simulink model "sim_battery_system"  (R2018b)
settings: Solver=FixedStepDiscrete  StartTime=0.0  StopTime=SimPara.t_sim  FixedStep=SimPara.t_step  RelTol=1e-3
undefined symbols (not defined in the file or in its folder): A, BatPara, i, LSAPara, p, SimPara, SysPara, x2_cal, x3_cal, x_cal
libraries: simulink x14, dspstat3 x4, dspindex x1
(part 1 of 4)
Description:
  | A simulation framework for lithium-ion battery systems.
  | Refer to https://github.com/TUMFTM/sim_battery_system for futher information.
  | 
  | Authors:
  | 
  | Christoph Reiter (christoph.reiter@tum.de)
  | Johannes Dirnecker
  | Leo Wildfeuer
  | André Thomaser
  | Thilo Krahl
  | Sebastian Huber
  | Thilo Wurster
  | 
  | Created at:
  | 
  | Institute of Automotive Technology
  | Department of Mechanical Engineering
  | Technical University of Munich
settings Model: SimulationMode=accelerator  NumberOfSteps=300  Creator=Christoph Reiter  LastModifiedBy=gu74niw
settings SolverCC: AutoInsertRateTranBlk=on  InsertRTBMode=Always
settings DataIOCC: LimitDataPoints=on  MaxDataPoints=1  SaveFormat=Structure  SaveOutput=off  SignalLogging=off  DSMLogging=off  SaveTime=off
settings OptimizationCC: DefaultParameterBehavior=Inlined  UseFloatMulNetSlope=on  InlineInvariantSignals=on  EfficientFloat2IntCast=on  LifeSpan=inf
settings DebuggingCC: ReadBeforeWriteMsg=DisableAll  WriteAfterWriteMsg=DisableAll  WriteAfterReadMsg=DisableAll  AlgebraicLoopMsg=error  SaveWithParameterizedLinksMsg=none  UnderspecifiedInitializationDetection=Classic  MultiTaskDSMMsg=none  MultiTaskCondExecSysMsg=warning  MultiTaskRateTransMsg=warning  SingleTaskRateTransMsg=warning  UniqueDataStoreMsg=error  AllowSymbolicDim=off  StrictBusMsg=ErrorOnBusTreatedAsVector  SFUnexpectedBacktrackingDiag=warning  SFNoUnconditionalDefaultTransitionDiag=warning  SFExecutionAtInitializationDiag=none
settings HardwareCC: ProdBitPerPointer=32  ProdBitPerSizeT=32  ProdBitPerPtrDiffT=32  ProdLargestAtomicFloat=None  ProdIntDivRoundTo=Undefined  ProdEndianess=Unspecified  ProdWordSize=32  ProdHWDeviceType=32-bit Generic  TargetBitPerPointer=64  TargetBitPerSizeT=64  TargetBitPerPtrDiffT=64  TargetLongLongMode=on  TargetIntDivRoundTo=Zero  TargetEndianess=LittleEndian  TargetWordSize=64  TargetHWDeviceType=MATLAB Host
settings ModelReferenceCC: UpdateModelReferenceTargets=IfOutOfDate  EnableParallelModelReferenceBuilds=on  ParallelModelReferenceMATLABWorkerInit=Load Top Model  PropagateSignalLabelsOutOfModel=off
settings SFSimCC: SFSimEcho=off  SimUseLocalCustomCode=off
settings RTWCC: RTWUseLocalCustomCode=off  Toolchain=Microsoft Visual C++ 2015 v14.0 | nmake (64-bit Windows)  BuildConfiguration=Faster Runs
settings CodeAppCC: ForceParamTrailComments=on  StateflowObjectComments=on  MATLABSourceComments=on
settings GRTTargetCC: GeneratePreprocessorConditionals=Disable all  MatFileLogging=off  SupportNonFinite=off
settings ConfigComp: CovMetricSettings=dw  CovHtmlReporting=on  CovSaveCumulativeToWorkspaceVar=on  CovSaveSingleToWorkspaceVar=on  CovExternalEMLEnable=off  CovSFcnEnable=off

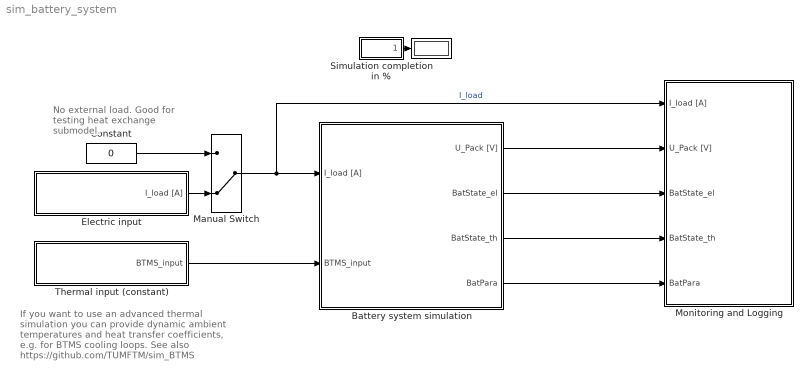
== system sim_battery_system ==
  note: No external load. Good for
      | testing heat exchange submodel.
  note: If you want to use an advanced thermal simulation
      | you can provide dynamic ambient temperatures
      | and heat transfer coefficients, e.g. for BTMS cooling
      | loops.
      | See also https://github.com/TUMFTM/sim_BTMS
  "\t\t      Simulation completion in %\t" : Subsystem
  " " : Display
      settings: Format=bank
  Battery system simulation : Subsystem  TreatAsAtomicUnit=on
  Constant : Constant  Value=0
  Electric input : Subsystem
  Manual Switch : ManualSwitch  CurrentSetting=0
  Monitoring and Logging : Subsystem
  Thermal input (constant) : Subsystem
  wires:
  "\t\t      Simulation completion in %\t"/1(" ") -> " "/1
  Manual Switch/1 -> Monitoring and Logging/1(I_load [A]), Battery system simulation/1(I_load [A])  "I_load"
  Thermal input (constant)/1(BTMS_input) -> Battery system simulation/2(BTMS_input)
  Battery system simulation/1(U_Pack [V]) -> Monitoring and Logging/2(U_Pack [V])
  Battery system simulation/2(BatState_el) -> Monitoring and Logging/3(BatState_el)
  Battery system simulation/3(BatState_th) -> Monitoring and Logging/4(BatState_th)
  Battery system simulation/4(BatPara) -> Monitoring and Logging/5(BatPara)
  Electric input/1(I_load [A]) -> Manual Switch/2
  Constant/1 -> Manual Switch/1

== system sim_battery_system/		      Simulation completion in %	 ==
  note: Determine simulation completion
  Clock : Clock
  Divide : Product  Inputs=*/
  max. Simulaton Time : Constant  Value=SimPara.t_sim
  to % : Gain  Gain=100
  " " : Outport
  wires:
  max. Simulaton Time/1 -> Divide/2
  Clock/1 -> Divide/1
  Divide/1 -> to %/1
  to %/1 -> " "/1

== system sim_battery_system/Battery system simulation ==
  I_load [A] : Inport
  BTMS_input : Inport  Port=2
  Electrical Submodel : Subsystem
  Save BatState_el of last time-step : Subsystem
  Save BatState_th of last time-step : Subsystem
  Static and dynamic LIB parameters : Subsystem
  Thermal Submodel : Subsystem
  U_Pack [V] : Outport
  BatState_el : Outport  Port=2
  BatState_th : Outport  Port=3
  BatPara : Outport  Port=4
  wires:
  Static and dynamic LIB parameters/1(BatPara) -> Electrical Submodel/2(BatPara), Thermal Submodel/4(BatPara), BatPara/1
  Electrical Submodel/1(BatState_el) -> BatState_el/1, Save BatState_el of last time-step/1(BatState_el), Thermal Submodel/3(BatState_el)
  I_load [A]/1 -> Electrical Submodel/1(I_Pack [A])
  Electrical Submodel/2(U_Pack [V]) -> U_Pack [V]/1
  Save BatState_el of last time-step/1(BatState_el_in) -> Static and dynamic LIB parameters/2(BatState_el_in), Electrical Submodel/3(BatState_in)
  Thermal Submodel/1(BatState_th) -> BatState_th/1, Save BatState_th of last time-step/1(BatState_th)
  Save BatState_th of last time-step/1(Bat_State_th_in) -> Thermal Submodel/1(BatState_th_in), Static and dynamic LIB parameters/1(BatState_th_in)
  BTMS_input/1 -> Thermal Submodel/2(BTMS_input)

== system sim_battery_system/Electric input ==
  note: Dummy load cycle. Scaled from cell measurement, so U_terminal
      | has nothing to do with the battery system you may specify.
  Demux : Demux  Outputs=2
  From Workspace : FromWorkspace  VariableName=load_cycle  SampleTime=0  OutputAfterFinalValue=Setting to zero
  Terminator : Terminator
  I_load [A] : Outport  Unit=A
  wires:
  From Workspace/1 -> Demux/1
  Demux/1 -> Terminator/1  "U_terminal"
  Demux/2 -> I_load [A]/1  "I_load"

== system sim_battery_system/Monitoring and Logging ==
  I_load [A] : Inport
  U_Pack [V] : Inport  Port=2
  BatState_el : Inport  Port=3
  BatState_th : Inport  Port=4
  BatPara : Inport  Port=5
  Constant : Constant  Value=SimPara.LoggingOutput
  Load Spectrum Analysis : Subsystem  Variant=on  VariantControl=Variant1
  Logging of Variables : Subsystem
  Temperature Sensor Simulation : Subsystem
  wires:
  I_load [A]/1 -> Logging of Variables/1(I_load [A])
  U_Pack [V]/1 -> Logging of Variables/2(U_Pack [A])
  BatState_el/1 -> Logging of Variables/3(BatState_el), Load Spectrum Analysis/1("BatState_el ")
  BatState_th/1 -> Temperature Sensor Simulation/1(bat_state_th_in)
  BatPara/1 -> Load Spectrum Analysis/3("BatPara ")
  Constant/1 -> Logging of Variables/Enable
  Temperature Sensor Simulation/1(bat_state_th_out) -> Load Spectrum Analysis/2("BatState_th ")

== system sim_battery_system/Thermal input (constant) ==
  Bus Creator : BusCreator  Inputs=2
  Constant : Constant  Value=SysPara.thermal.T_cell_ambient
  Constant1 : Constant  Value=SysPara.thermal.alpha_cell_ambient
  BTMS_input : Outport
  wires:
  Constant1/1 -> Bus Creator/2  "alpha_cell_ambient"
  Constant/1 -> Bus Creator/1  "T_cell_ambient"
  Bus Creator/1 -> BTMS_input/1  "BTMS_input"

== system sim_battery_system/Battery system simulation/Electrical Submodel ==
  note: Delay resulting balancing current for one step to avoid algebraic loop
  I_Pack [A] : Inport
  BatPara : Inport  Port=2
  BatState_in : Inport  Port=3
  Bus Creator1 : BusCreator  Inputs=8
  Cell Balancing : Subsystem
  Electric potential (single cell) : Subsystem
  Ohmic voltage drop and compensating currents in parallel connections : Subsystem
  Unit Delay4 : UnitDelay  InitialCondition=zeros(SysPara.p,SysPara.s)  SampleTime=-1
  Voltage of battery system : Subsystem
  dt : Subsystem
  BatState_el : Outport
  U_Pack [V] : Outport  Port=2
  wires:
  I_Pack [A]/1 -> Cell Balancing/1(I_Pack [A]), Ohmic voltage drop and compensating currents in parallel connections/2(I_Pack [A])
  Unit Delay4/1 -> Ohmic voltage drop and compensating currents in parallel connections/1(I_Balancing_in [A])  "I_Balancing_in [A]"
  Ohmic voltage drop and compensating currents in parallel connections/1(U_Cell [V]) -> Bus Creator1/1, Voltage of battery system/1(U_Cells [V]), Cell Balancing/2(U_Cell [V])
  Ohmic voltage drop and compensating currents in parallel connections/2(I_Cell [A]) -> Bus Creator1/2
  Ohmic voltage drop and compensating currents in parallel connections/3(U_R [V]) -> Bus Creator1/3
  Cell Balancing/1(I_Balancing [A]) -> Unit Delay4/1
  Voltage of battery system/1(U_Pack [V]) -> U_Pack [V]/1
  Bus Creator1/1 -> BatState_el/1  "BatState_el"
  BatPara/1 -> Ohmic voltage drop and compensating currents in parallel connections/3(BatPara), Electric potential (single cell)/1(BatPara)
  Electric potential (single cell)/1(U_Potential) -> Ohmic voltage drop and compensating currents in parallel connections/4(U_Potential [V]), Bus Creator1/4
  dt/1(dt [s]) -> Electric potential (single cell)/2(dt)
  BatState_in/1 -> Electric potential (single cell)/3(BatState_in)
  Electric potential (single cell)/2(SOC) -> Bus Creator1/5
  Electric potential (single cell)/3(U_OCV) -> Bus Creator1/6
  Electric potential (single cell)/4(U_Hysteresis) -> Bus Creator1/7
  Electric potential (single cell)/5(U_RC) -> Bus Creator1/8

== system sim_battery_system/Battery system simulation/Save BatState_el of last time-step ==
  note: Delay system state variables by one step to avoid algebraic loop.
      | We need these for the parameter lookup-tables
  BatState_el : Inport
  Bus Creator : BusCreator  Inputs=4
  Bus Creator2 : BusCreator  Inputs=4
  Bus Selector : BusSelector  OutputSignals=U_RC1 [V],U_RC2 [V],U_RC3 [V],U_RC4 [V]
  Bus Selector1 : BusSelector  OutputSignals=SOC,U_Hysteresis [V],I_cell [A],U_RC [V]
  Unit Delay : UnitDelay  InitialCondition=SysPara.BatStateInit.electrical.SOC  SampleTime=-1
  Unit Delay1 : UnitDelay  InitialCondition=SysPara.BatStateInit.electrical.U_hyst  SampleTime=-1
  Unit Delay2 : UnitDelay  InitialCondition=SysPara.BatStateInit.electrical.U_RC1  SampleTime=-1
  Unit Delay3 : UnitDelay  InitialCondition=SysPara.BatStateInit.electrical.U_RC2  SampleTime=-1
  Unit Delay4 : UnitDelay  InitialCondition=SysPara.BatStateInit.electrical.I_cell  SampleTime=-1
  Unit Delay5 : UnitDelay  InitialCondition=SysPara.BatStateInit.electrical.U_RC3  SampleTime=-1
  Unit Delay6 : UnitDelay  InitialCondition=SysPara.BatStateInit.electrical.U_RC4  SampleTime=-1
  BatState_el_in : Outport
  wires:
  Bus Selector1/2 -> Unit Delay1/1  "<U_Hysteresis [V]>"
  Unit Delay4/1 -> Bus Creator2/3  "I_cell [A]"
  Bus Selector1/3 -> Unit Delay4/1  "<I_cell [A]>"
  Unit Delay1/1 -> Bus Creator2/2  "U_Hysteresis [V]"
  Bus Selector1/1 -> Unit Delay/1  "<SOC>"
  Unit Delay/1 -> Bus Creator2/1  "SOC"
  Bus Creator2/1 -> BatState_el_in/1  "BatState_el_in"
  BatState_el/1 -> Bus Selector1/1
  Bus Selector1/4 -> Bus Selector/1  "<U_RC [V]>"
  Bus Selector/1 -> Unit Delay2/1  "<U_RC1 [V]>"
  Bus Selector/2 -> Unit Delay3/1  "<U_RC2 [V]>"
  Bus Selector/3 -> Unit Delay5/1  "<U_RC3 [V]>"
  Bus Selector/4 -> Unit Delay6/1  "<U_RC4 [V]>"
  Unit Delay6/1 -> Bus Creator/4  "U_RC4 [V]"
  Unit Delay5/1 -> Bus Creator/3  "U_RC3 [V]"
  Unit Delay3/1 -> Bus Creator/2  "U_RC2 [V]"
  Unit Delay2/1 -> Bus Creator/1  "U_RC1 [V]"
  Bus Creator/1 -> Bus Creator2/4  "U_RC"

== system sim_battery_system/Battery system simulation/Save BatState_th of last time-step ==
  note: Delay system state variables by one step to avoid algebraic loop.
      | We need these for the parameter lookup-tables
  BatState_th : Inport
  Bus Creator1 : BusCreator  Inputs=1
  Bus Selector : BusSelector  OutputSignals=T_cell [°C]
  Unit Delay1 : UnitDelay  InitialCondition=SysPara.BatStateInit.thermal.T_cell  SampleTime=-1
  Bat_State_th_in : Outport
  wires:
  Unit Delay1/1 -> Bus Creator1/1  "T_cell [°C]"
  Bus Selector/1 -> Unit Delay1/1  "<T_cell [°C]>"
  Bus Creator1/1 -> Bat_State_th_in/1  "Bat_State_th_in"
  BatState_th/1 -> Bus Selector/1

== system sim_battery_system/Battery system simulation/Static and dynamic LIB parameters ==
  BatState_th_in : Inport
  BatState_el_in : Inport  Port=2
  LIB Parameter Look-Ups : Subsystem
  Statistic Cell Deviations : Subsystem
  BatPara : Outport
  wires:
  LIB Parameter Look-Ups/1(BatPara_el_uniform) -> Statistic Cell Deviations/1("BatPara_el_uniform ")
  Statistic Cell Deviations/1(BatPara) -> BatPara/1  "BatPara"
  BatState_el_in/1 -> LIB Parameter Look-Ups/2(BatState_el_in)
  BatState_th_in/1 -> LIB Parameter Look-Ups/1(BatState_th_in)

== system sim_battery_system/Battery system simulation/Thermal Submodel ==
  note: Total cell heat generation:
      |
      | PQ_cell = PQ_cell,irr + PQ_cell,rev
  BatState_th_in : Inport
  BTMS_input : Inport  Port=2
  BatState_el : Inport  Port=3
  BatPara : Inport  Port=4
  Add : Sum
  Bus Creator : BusCreator  Inputs=6
  Bus Selector : BusSelector  OutputSignals=U_R [V],U_RC [V],I_cell [A]
  Bus Selector3 : BusSelector  OutputSignals=alpha_cell_ambient,T_cell_ambient
  Bus Selector4 : BusSelector  OutputSignals=T_cell [°C]
  Cell heat transport and heat dissipation : Subsystem
  Constant : Constant  Value=SimPara.thermal_sim_enable
  Irreversible heat generation : Subsystem
  Reversible heat generation : Subsystem
  BatState_th : Outport
  wires:
  Bus Selector3/2 -> Cell heat transport and heat dissipation/5(T_cell_ambient), Bus Creator/5  "<T_cell_ambient>"
  Add/1 -> Cell heat transport and heat dissipation/1(PQ_cell), Bus Creator/1  "PQ_cell [W]"
  Bus Creator/1 -> BatState_th/1  "BatState_th"
  Bus Selector3/1 -> Cell heat transport and heat dissipation/4(alpha_cell_ambient), Bus Creator/6  "<alpha_cell_ambient>"
  Irreversible heat generation/1(PQ_cell,irr [W]) -> Add/1
  Reversible heat generation/1(PQ_cell,rev [W]) -> Add/2
  BatPara/1 -> Cell heat transport and heat dissipation/2(BatPara), Reversible heat generation/3(BatPara)
  BatState_el/1 -> Bus Selector/1
  Bus Selector/2 -> Irreversible heat generation/2(U_RC)  "<U_RC [V]>"
  Bus Selector/3 -> Reversible heat generation/1(I_Cells [A]), Irreversible heat generation/3(I_Cells [A])  "<I_cell [A]>"
  Bus Selector/1 -> Irreversible heat generation/1(U_R [V])  "<U_R [V]>"
  BTMS_input/1 -> Bus Selector3/1
  BatState_th_in/1 -> Bus Selector4/1
  Bus Selector4/1 -> Reversible heat generation/2(T_Cells [°C]), Cell heat transport and heat dissipation/3(T_cell_in)  "<T_cell [°C]>"
  Cell heat transport and heat dissipation/1(T_cell [°C]) -> Bus Creator/2
  Constant/1 -> Cell heat transport and heat dissipation/Enable
  Cell heat transport and heat dissipation/3(PQ_transfer [W]) -> Bus Creator/4
  Cell heat transport and heat dissipation/2(PQ_ambient [W]) -> Bus Creator/3

== system sim_battery_system/Monitoring and Logging/Load Spectrum Analysis ==
  "BatState_el " : Inport
  "BatState_th " : Inport  Port=2
  "BatPara " : Inport  Port=3
  Load Spectrum Analysis OFF : Subsystem  VariantControl=SimPara.LoadSpectra_enable == 0
  Load Spectrum Analysis ON : Subsystem  VariantControl=SimPara.LoadSpectra_enable == 1

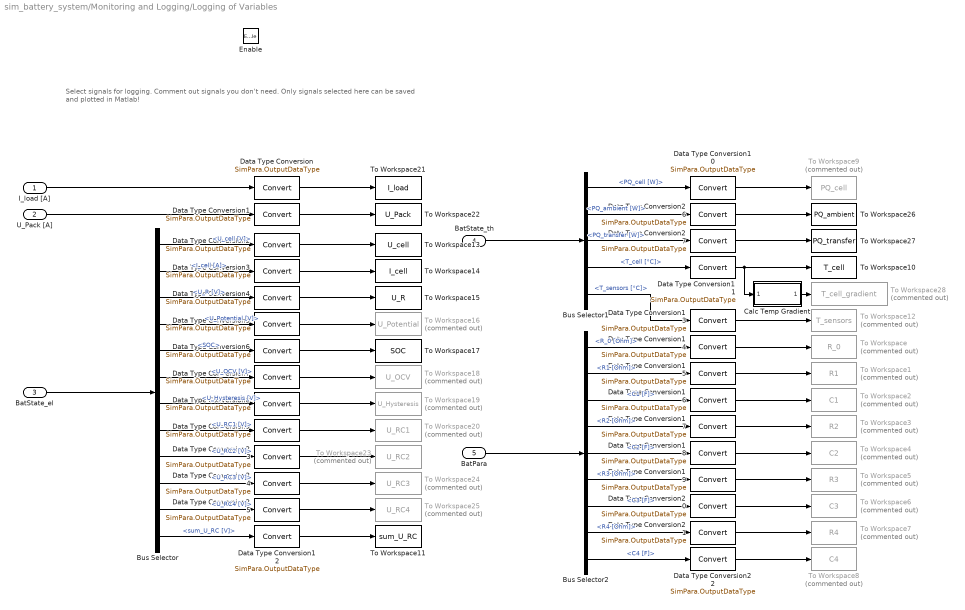
== system sim_battery_system/Monitoring and Logging/Logging of Variables ==
  note: Select signals for logging. Comment out signals you don't need.
      | Only signals selected here can be saved and plotted in Matlab!
  I_load [A] : Inport
  U_Pack [A] : Inport  Port=2
  BatState_el : Inport  Port=3
  BatState_th : Inport  Port=4
  BatPara : Inport  Port=5
  Enable : EnablePort
  Bus Selector : BusSelector  OutputSignals=U_cell [V],I_cell [A],U_R [V],U_Potential [V],SOC,U_OCV [V],U_Hysteresis [V],U_RC [V].U_RC1 [V],U_RC [V].U_RC2 [V],U_RC [V].U_RC3 [V],U_RC [V].U_RC4 [V],U_RC [V].sum_U_RC [V]
  Bus Selector1 : BusSelector  OutputSignals=PQ_cell [W],PQ_ambient [W],PQ_transfer [W],T_cell [°C],T_sensors [°C]
  Bus Selector2 : BusSelector  OutputSignals=electrical.R_0 [Ohm],electrical.R1 [Ohm],electrical.C1 [F],electrical.R2 [Ohm],electrical.C2 [F],electrical.R3 [Ohm],electrical.C3 [F],electrical.R4 [Ohm],electrical.C4 [F]
  Calc Temp Gradient : Subsystem
  Data Type Conversion{,1..27} (28 alike) : DataTypeConversion  OutDataTypeStr=SimPara.OutputDataType
  To Workspace : ToWorkspace  Commented=on  VariableName=R_0  SaveFormat=Timeseries  SampleTime=-1
      settings: Decimation=SimPara.OutputDecimation
  To Workspace1 : ToWorkspace  Commented=on  VariableName=R1  SaveFormat=Timeseries  SampleTime=-1
      settings: Decimation=SimPara.OutputDecimation
  To Workspace10 : ToWorkspace  VariableName=T_cell  SaveFormat=Timeseries  SampleTime=-1
      settings: Decimation=SimPara.OutputDecimation
  To Workspace11 : ToWorkspace  VariableName=sum_U_RC  SaveFormat=Timeseries  SampleTime=-1
      settings: Decimation=SimPara.OutputDecimation
  To Workspace12 : ToWorkspace  Commented=on  VariableName=T_sensors  SaveFormat=Timeseries  SampleTime=-1
      settings: Decimation=SimPara.OutputDecimation
  To Workspace13 : ToWorkspace  VariableName=U_cell  SaveFormat=Timeseries  SampleTime=-1
      settings: Decimation=SimPara.OutputDecimation
  To Workspace14 : ToWorkspace  VariableName=I_cell  SaveFormat=Timeseries  SampleTime=-1
      settings: Decimation=SimPara.OutputDecimation
  To Workspace15 : ToWorkspace  VariableName=U_R  SaveFormat=Timeseries  SampleTime=-1
      settings: Decimation=SimPara.OutputDecimation
  To Workspace16 : ToWorkspace  Commented=on  VariableName=U_Potential  SaveFormat=Timeseries  SampleTime=-1
      settings: Decimation=SimPara.OutputDecimation
  To Workspace17 : ToWorkspace  VariableName=SOC  SaveFormat=Timeseries  SampleTime=-1
      settings: Decimation=SimPara.OutputDecimation
  To Workspace18 : ToWorkspace  Commented=on  VariableName=U_OCV  SaveFormat=Timeseries  SampleTime=-1
      settings: Decimation=SimPara.OutputDecimation
  To Workspace19 : ToWorkspace  Commented=on  VariableName=U_Hysteresis  SaveFormat=Timeseries  SampleTime=-1
      settings: Decimation=SimPara.OutputDecimation
  To Workspace2 : ToWorkspace  Commented=on  VariableName=C1  SaveFormat=Timeseries  SampleTime=-1
      settings: Decimation=SimPara.OutputDecimation
  To Workspace20 : ToWorkspace  Commented=on  VariableName=U_RC1  SaveFormat=Timeseries  SampleTime=-1
      settings: Decimation=SimPara.OutputDecimation
  To Workspace21 : ToWorkspace  VariableName=I_load  SaveFormat=Timeseries  SampleTime=-1
      settings: Decimation=SimPara.OutputDecimation
  To Workspace22 : ToWorkspace  VariableName=U_Pack  SaveFormat=Timeseries  SampleTime=-1
      settings: Decimation=SimPara.OutputDecimation
  To Workspace23 : ToWorkspace  Commented=on  VariableName=U_RC2  SaveFormat=Timeseries  SampleTime=-1
      settings: Decimation=SimPara.OutputDecimation
  To Workspace24 : ToWorkspace  Commented=on  VariableName=U_RC3  SaveFormat=Timeseries  SampleTime=-1
      settings: Decimation=SimPara.OutputDecimation
  To Workspace25 : ToWorkspace  Commented=on  VariableName=U_RC4  SaveFormat=Timeseries  SampleTime=-1
      settings: Decimation=SimPara.OutputDecimation
  To Workspace26 : ToWorkspace  VariableName=PQ_ambient  SaveFormat=Timeseries  SampleTime=-1
      settings: Decimation=SimPara.OutputDecimation
  To Workspace27 : ToWorkspace  VariableName=PQ_transfer  SaveFormat=Timeseries  SampleTime=-1
      settings: Decimation=SimPara.OutputDecimation
  To Workspace28 : ToWorkspace  Commented=on  VariableName=T_cell_gradient  SaveFormat=Timeseries  SampleTime=-1
      settings: Decimation=SimPara.OutputDecimation
  To Workspace3 : ToWorkspace  Commented=on  VariableName=R2  SaveFormat=Timeseries  SampleTime=-1
      settings: Decimation=SimPara.OutputDecimation
  To Workspace4 : ToWorkspace  Commented=on  VariableName=C2  SaveFormat=Timeseries  SampleTime=-1
      settings: Decimation=SimPara.OutputDecimation
  To Workspace5 : ToWorkspace  Commented=on  VariableName=R3  SaveFormat=Timeseries  SampleTime=-1
      settings: Decimation=SimPara.OutputDecimation
  To Workspace6 : ToWorkspace  Commented=on  VariableName=C3  SaveFormat=Timeseries  SampleTime=-1
      settings: Decimation=SimPara.OutputDecimation
  To Workspace7 : ToWorkspace  Commented=on  VariableName=R4  SaveFormat=Timeseries  SampleTime=-1
      settings: Decimation=SimPara.OutputDecimation
  To Workspace8 : ToWorkspace  Commented=on  VariableName=C4  SaveFormat=Timeseries  SampleTime=-1
      settings: Decimation=SimPara.OutputDecimation
  To Workspace9 : ToWorkspace  Commented=on  VariableName=PQ_cell  SaveFormat=Timeseries  SampleTime=-1
      settings: Decimation=SimPara.OutputDecimation
  wires:
  Data Type Conversion2/1 -> To Workspace13/1
  Data Type Conversion6/1 -> To Workspace17/1
  Data Type Conversion8/1 -> To Workspace19/1
  U_Pack [A]/1 -> Data Type Conversion1/1
  Bus Selector/11 -> Data Type Conversion25/1  "<U_RC4 [V]>"
  Bus Selector/5 -> Data Type Conversion6/1  "<SOC>"
  Bus Selector/10 -> Data Type Conversion24/1  "<U_RC3 [V]>"
  Bus Selector/12 -> Data Type Conversion12/1  "<sum_U_RC [V]>"
  Bus Selector/3 -> Data Type Conversion4/1  "<U_R [V]>"
  Bus Selector/7 -> Data Type Conversion8/1  "<U_Hysteresis [V]>"
  Data Type Conversion23/1 -> To Workspace23/1
  Data Type Conversion/1 -> To Workspace21/1
  Bus Selector/2 -> Data Type Conversion3/1  "<I_cell [A]>"
  Bus Selector/1 -> Data Type Conversion2/1  "<U_cell [V]>"
  Bus Selector/6 -> Data Type Conversion7/1  "<U_OCV [V]>"
  Data Type Conversion24/1 -> To Workspace24/1
  Data Type Conversion3/1 -> To Workspace14/1
  Data Type Conversion5/1 -> To Workspace16/1
  Data Type Conversion9/1 -> To Workspace20/1
  Data Type Conversion4/1 -> To Workspace15/1
  Data Type Conversion1/1 -> To Workspace22/1
  Data Type Conversion7/1 -> To Workspace18/1
  Data Type Conversion25/1 -> To Workspace25/1
  Bus Selector/8 -> Data Type Conversion9/1  "<U_RC1 [V]>"
  Data Type Conversion12/1 -> To Workspace11/1
  Bus Selector/4 -> Data Type Conversion5/1  "<U_Potential [V]>"
  Bus Selector/9 -> Data Type Conversion23/1  "<U_RC2 [V]>"
  I_load [A]/1 -> Data Type Conversion/1
  BatState_el/1 -> Bus Selector/1
  Calc Temp Gradient/1(T_cell_gradient) -> To Workspace28/1
  Data Type Conversion19/1 -> To Workspace5/1
  Data Type Conversion17/1 -> To Workspace3/1
  Bus Selector2/4 -> Data Type Conversion17/1  "<R2 [Ohm]>"
  Bus Selector1/1 -> Data Type Conversion10/1  "<PQ_cell [W]>"
  Bus Selector2/9 -> Data Type Conversion22/1  "<C4 [F]>"
  Data Type Conversion14/1 -> To Workspace/1
  BatPara/1 -> Bus Selector2/1
  Bus Selector2/3 -> Data Type Conversion16/1  "<C1 [F]>"
  Data Type Conversion15/1 -> To Workspace1/1
  Bus Selector2/7 -> Data Type Conversion20/1  "<C3 [F]>"
  Data Type Conversion13/1 -> To Workspace12/1
  Bus Selector2/5 -> Data Type Conversion18/1  "<C2 [F]>"
  BatState_th/1 -> Bus Selector1/1
  Bus Selector2/1 -> Data Type Conversion14/1  "<R_0 [Ohm]>"
  Data Type Conversion22/1 -> To Workspace8/1
  Data Type Conversion10/1 -> To Workspace9/1
  Data Type Conversion11/1 -> To Workspace10/1, Calc Temp Gradient/1(T_cell)
  Bus Selector1/4 -> Data Type Conversion11/1  "<T_cell [°C]>"
  Data Type Conversion18/1 -> To Workspace4/1
  Bus Selector2/2 -> Data Type Conversion15/1  "<R1 [Ohm]>"
  Data Type Conversion16/1 -> To Workspace2/1
  Bus Selector1/3 -> Data Type Conversion27/1  "<PQ_transfer [W]>"
  Bus Selector1/5 -> Data Type Conversion13/1  "<T_sensors [°C]>"
  Bus Selector1/2 -> Data Type Conversion26/1  "<PQ_ambient [W]>"
  Data Type Conversion20/1 -> To Workspace6/1
  Data Type Conversion21/1 -> To Workspace7/1
  Bus Selector2/6 -> Data Type Conversion19/1  "<R3 [Ohm]>"
  Data Type Conversion26/1 -> To Workspace26/1
  Bus Selector2/8 -> Data Type Conversion21/1  "<R4 [Ohm]>"
  Data Type Conversion27/1 -> To Workspace27/1

== system sim_battery_system/Monitoring and Logging/Temperature Sensor Simulation ==
  bat_state_th_in : Inport
  Bus Selector : BusSelector  OutputSignals=T_cell [°C]
  Enable/disable temperature sensors : Subsystem  Variant=on
  Rebuild bus structure : Subsystem
  bat_state_th_out : Outport
  wires:
  bat_state_th_in/1 -> Bus Selector/1, Rebuild bus structure/2(Bat_state_th_in)
  Bus Selector/1 -> Enable/disable temperature sensors/1(T_cell)  "<T_cell [°C]>"
  Enable/disable temperature sensors/1(T_sensors [°C]) -> Rebuild bus structure/1(T_sensors)
  Rebuild bus structure/1(bat_state_th_out) -> bat_state_th_out/1

== system sim_battery_system/Battery system simulation/Electrical Submodel/Cell Balancing ==
  note: The balancing function is only active if the following three conditions are met:
  note: -> Da zu einem Auswertungszeitpunkt das Stattfinden von Balancing auf Basis der Klemmenspannungen der Zellen bestimmt wird und die Balancing-Ströme der Zellen ebenfalls über deren Klemmenspannungen berechnet werden, können bei Balancing-Auftritt diese Balancing-Ströme erst zum nächsten Auswertungszeitpunkt für die Berechnung der neuen Klemmenspannungen und Strombelastungen der Zellen verwendet werden
      | -> Dadurch wird ein Fehler gemacht, der im diskreten Modell jedoch unvermeidbar ist
  note: Simple dissipative balancing.
      | Attention: For maximum flexibility of the model it is assumed every cell has it's own balancing resistor. Of course, in a parallel connection the equalisation effects allow the cells to share one balancing resistor. Therefore, a parallel connection of 5 cells with a balancing resistor of 33 Ohm would be set up like this: SysPara.Balancing.R = 33/5
  note: Condition 1: Terminal voltages of all cells in the battery pack >= Balancing.U_Limit
  note: The lowest terminal voltage of all cells in the battery pack always serves as reference.
      | à If the voltage difference between the terminal voltage of a cell and the reference voltage is greater than Balancing.U_Delta, this cell is connected to its balancing resistor.
      | à Condition for balancing: U_cell - reference voltage > Balancing.U_Delta
      | à It is not enough, if the voltage difference is equal to Balancing.U_Delta à The reason for this is that otherwise, with Balancing.U_Delta = 0, the cells with the lowest terminal voltage would also have their balancing resistors switched on.
  note: Determination of the balancing currents of the cells:
      | à The balancing current is the current that loads the cell when the balancing resistor is switched on.
      | à Calculation via the terminal voltages of the cells and via the balancing resistances of the cells using Ohm's law
      | à A negative sign must be considered in the equation because the balancing current discharges a cell and currents are defined negatively in the battery pack model for discharging.
      | I_Balancing = - U_cell / Balancing.R
  note: Condition 2: Amount of the external current load of the battery pack <= Balancing.I_Limit
  note: Condition 3: Simulation time >= Balancing.t_Start
  I_Pack [A] : Inport
  U_Cell [V] : Inport  Port=2
  Abs : Abs
  Clock : Clock
  Constant : Constant  Value=SysPara.Balancing.R  VectorParams1D=off
  Constant1 : Constant  Value=SysPara.Balancing.U_Delta  VectorParams1D=off
  Constant2 : Constant  Value=SysPara.Balancing.U_Limit  VectorParams1D=off
  Constant3 : Constant  Value=SysPara.Balancing.I_Limit  VectorParams1D=off
  Constant4 : Constant  Value=SysPara.Balancing.t_Start
  Divide : Product  Inputs=/*
  Gain : Gain  Gain=-1  OutDataTypeStr=double
  Minimum : dspstat3/Minimum  operation=minimum  fcn=Value  indexBase=One  operateOver=Entire input  Dimension=1  InputProcessing=Columns as channels (frame based)  reset=None  roiEnable=off  roiType=Rectangles  roiPortion=Entire ROI  roiOutput=Individual statistics for each ROI  roiFlag=off  roundingMode=Floor  overflowMode=off
      settings: SourceProductName=DSP System Toolbox  SourceProductBaseCode=DS
  Product : Product  Inputs=5
  Relational Operator : RelationalOperator  Operator=>  OutDataTypeStr=boolean  RndMeth=Simplest
  Relational Operator1 : RelationalOperator  OutDataTypeStr=boolean  RndMeth=Simplest
  Relational Operator2 : RelationalOperator  Operator=<=  OutDataTypeStr=boolean  RndMeth=Simplest
  Relational Operator3 : RelationalOperator  OutDataTypeStr=boolean  RndMeth=Simplest
  Subtract : Sum  Inputs=+-
  I_Balancing [A] : Outport
  wires:
  U_Cell [V]/1 -> Minimum/1, Divide/2, Subtract/1
  Product/1 -> I_Balancing [A]/1  "I_Balancing [A]"
  Minimum/1 -> Relational Operator1/1, Subtract/2
  Constant/1 -> Divide/1
  Constant1/1 -> Relational Operator/2
  I_Pack [A]/1 -> Abs/1
  Constant3/1 -> Relational Operator2/2
  Clock/1 -> Relational Operator3/1
  Constant4/1 -> Relational Operator3/2
  Constant2/1 -> Relational Operator1/2
  Relational Operator3/1 -> Product/5
  Relational Operator2/1 -> Product/4
  Relational Operator1/1 -> Product/3
  Relational Operator/1 -> Product/2
  Divide/1 -> Gain/1
  Gain/1 -> Product/1
  Abs/1 -> Relational Operator2/1
  Subtract/1 -> Relational Operator/1

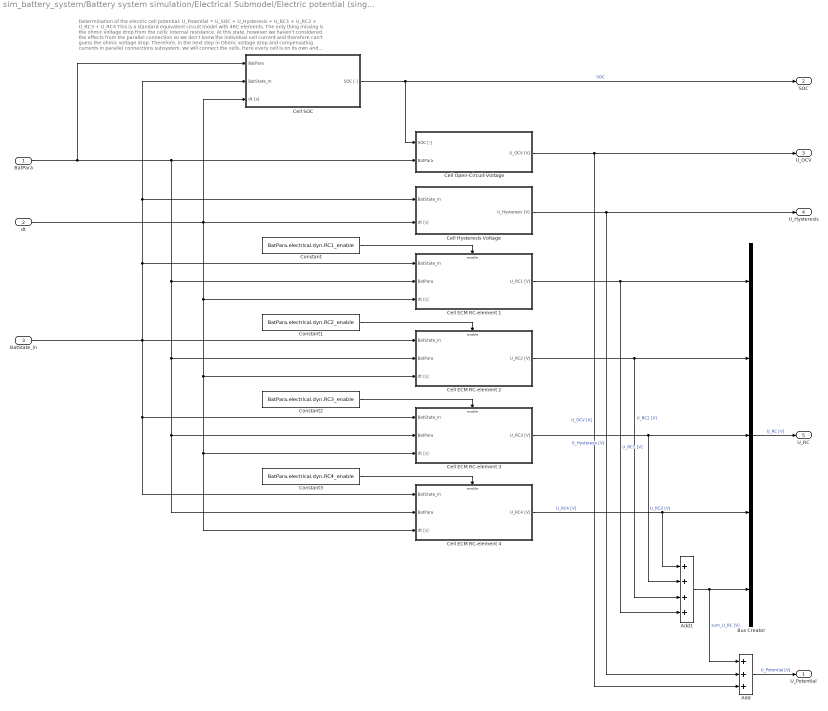
== system sim_battery_system/Battery system simulation/Electrical Submodel/Electric potential (single cell) ==
  note: Determination of the electric cell potential: U_Potential = U_SOC + U_Hysteresis + U_RC1 + U_RC2 + U_RC3 + U_RC4
      |
      | This is a standard equivalent circuit model with 4RC elements. The only thing missing is the ohmic voltage drop from the cells' internal resistance. At this state, however we haven't considered the effects from the parallel connection so we don't know the individual cell current and therefore can't guess the ohmic voltage drop. Therefore, in the next step in Ohmic voltage drop and compensating currents in parallel connections subsystem, we will connect the cells. Here every cell is on its own and doesn't interact with the other cells ins the syster (yet).
  BatPara : Inport
  dt : Inport  Port=2
  BatState_in : Inport  Port=3
  Add : Sum  Inputs=+++
  Add1 : Sum  Inputs=++++
  Bus Creator : BusCreator  Inputs=5
  Cell ECM RC-element 1 : Subsystem
  Cell ECM RC-element 2 : Subsystem
  Cell ECM RC-element 3 : Subsystem
  Cell ECM RC-element 4 : Subsystem
  Cell Hysteresis Voltage : Subsystem
  Cell Open-Circuit-Voltage : Subsystem
  Cell SOC : Subsystem
  Constant : Constant  Value=BatPara.electrical.dyn.RC1_enable
  Constant1 : Constant  Value=BatPara.electrical.dyn.RC2_enable
  Constant2 : Constant  Value=BatPara.electrical.dyn.RC3_enable
  Constant3 : Constant  Value=BatPara.electrical.dyn.RC4_enable
  U_Potential : Outport
  SOC : Outport  Port=2
  U_OCV : Outport  Port=3
  U_Hysteresis : Outport  Port=4
  U_RC : Outport  Port=5
  wires:
  BatState_in/1 -> Cell ECM RC-element 4/1(BatState_In), Cell ECM RC-element 3/1(BatState_In), Cell ECM RC-element 2/1(BatState_In), Cell Hysteresis Voltage/1(BatState_In), Cell SOC/2(BatState_In), Cell ECM RC-element 1/1(BatState_In)
  Cell ECM RC-element 1/1(U_RC1 [V]) -> Add1/4, Bus Creator/1  "U_RC1 [V]"
  Cell SOC/1(SOC [-]) -> Cell Open-Circuit-Voltage/1(SOC [-]), SOC/1  "SOC"
  Cell Open-Circuit-Voltage/1(U_OCV [V]) -> Add/3, U_OCV/1  "U_OCV [V]"
  dt/1 -> Cell ECM RC-element 4/3(dt [s]), Cell ECM RC-element 3/3(dt [s]), Cell ECM RC-element 2/3(dt [s]), Cell ECM RC-element 1/3(dt [s]), Cell SOC/3(dt [s]), Cell Hysteresis Voltage/2(dt [s])
  Cell ECM RC-element 2/1(U_RC2 [V]) -> Add1/3, Bus Creator/2  "U_RC2 [V]"
  BatPara/1 -> Cell Open-Circuit-Voltage/2(BatPara), Cell ECM RC-element 1/2(BatPara), Cell ECM RC-element 2/2(BatPara), Cell ECM RC-element 3/2(BatPara), Cell ECM RC-element 4/2(BatPara), Cell SOC/1(BatPara)
  Cell Hysteresis Voltage/1(U_Hysteresis [V]) -> Add/2, U_Hysteresis/1  "U_Hysteresis [V]"
  Add/1 -> U_Potential/1  "U_Potential [V]"
  Cell ECM RC-element 3/1(U_RC3 [V]) -> Add1/2, Bus Creator/3  "U_RC3 [V]"
  Cell ECM RC-element 4/1(U_RC4 [V]) -> Add1/1, Bus Creator/4  "U_RC4 [V]"
  Bus Creator/1 -> U_RC/1  "U_RC [V]"
  Add1/1 -> Add/1, Bus Creator/5  "sum_U_RC [V]"
  Constant/1 -> Cell ECM RC-element 1/Enable
  Constant1/1 -> Cell ECM RC-element 2/Enable
  Constant2/1 -> Cell ECM RC-element 3/Enable
  Constant3/1 -> Cell ECM RC-element 4/Enable

== system sim_battery_system/Battery system simulation/Electrical Submodel/Ohmic voltage drop and compensating currents in parallel connections ==
  note: Now it gets complicated… In this step the cells are connected in serial and parallel and the current distribution in the parallel connection as well as the compensating currents are calculated. The calculation makes heavy use of the matrix structure of the signals so many things happen at ones. Here follows a shot summary of what happens here.
      | Steps for determining the terminal voltages and current loads of the cells:
      | 1. Assumption of the interconnection mechanism of the cells: Cells are first connected in parallel to a network -> parallel cell networks are then connected in series
      | 2. Determination of the current loads of the cells connected in parallel, which consider the compensating currents, by means of a backward calculation using the terminal voltages of the cells and knowledge of the potentials and ohmic internal resistances of the cells.
      | 3. Terminal voltages of the cells in a parallel cell system = terminal voltage of the parallel cell system
      | 4. Calculation of the terminal voltage of a parallel cell system via a representative total current in the parallel cell system and via a substitute resistance of the parallel cell system using Ohm's law.
      | 5. For the representative total current in a parallel cell network, the information about the potentials of the cells in this network must be considered à This is possible via the short-circuit currents of the cells in this network.
      | 6. The further proportions of the representative total current in a parallel cell system refer to an occurring current load -> External current load of the battery pack, because this is present at each parallel cell system due to the assumed interconnection mechanism in the battery pack model, and balancing currents of the cells in this system.
      | 7. The equivalent resistance of a parallel cell composite results from the total resistances of the individual cells in this composite.
      |
      | Determination of the terminal voltages of the cells:
      | 1. short-circuit currents of the cells = U_Potential / R_0 (ohmic internal resistances of the cells)
      | è Short circuit current of a cell contains the information about the potential of the cell.
      | è Calculation background: The electrical equivalent circuit of a cell is simplified to the potential of the cell and the ohmic internal resistance of the cell à When the cell is short-circuited, the entire potential of the cell drops at the ohmic internal resistance of the cell.
      | 2. Addition of the short-circuit currents of the cells via cells connected in parallel
      | 3. Add I_load (external current load of the battery pack) to each parallel cell array.
      | 4. Adding of I_Balancing (see subsystem "Balancing") to the cells via parallel connected cells
      | 5. The sum of these currents gives the representative total current in each parallel cell system or the total current in each parallel cell system including consideration of the short circuits of the cells.
      | 6. For the simplified equivalent electrical circuit, which is used for the realization of the equalizing currents, the total resistance of a cell consists only of the ohmic internal resistance of the cell
      | è Determination of the equivalent resistance of a parallel cell network via parallel connection of the ohmic internal resistances of the cells in this network
      | è Add up the reciprocal values of the ohmic internal resistances of the cells via cells connected in parallel: 1/R_ges = 1/R_1 + 1/R_2 + ...
      | è Replacement resistance of a parallel cell network corresponds to the reciprocal value of the result
      | 7. Terminal voltage of a parallel cell system = total current in the parallel cell system including consideration of the short circuits of the cells * Replacement resistance of the parallel cell system = terminal voltage of each cell in the parallel cell system because cells connected in parallel have the same terminal voltage
      | è U_cell (terminal voltages of the cells) successfully calculated
      |
      | Determination of the current loads of the cells:
      | 1. U_R (ohmic voltage components of the cells) = U_cell - U_Potential
      | 2. I_cell (current loads of the cells) = U_R / R_0
      |
      | Result:
      | à I_cell considers the equalizing currents in a parallel cell array, which always ensure identical terminal voltages of the cells in this array -> Physical condition in a parallel cell array
      | à The short-circuit currents of the cells are included in the calculation so that the potentials of the cells can be considered when calculating the terminal voltage.
      | à For U_R = U_cell - U_Potential the potentials of the individual cells are calculated again.
      | à Sum of the current loads of the cells in a parallel cell network = External current load of the battery pack + Sum of the balancing currents of the cells in this network -> Correct physical correlation
  I_Balancing_in [A] : Inport
  I_Pack [A] : Inport  Port=2
  BatPara : Inport  Port=3
  U_Potential [V] : Inport  Port=4
  Add : Sum  Inputs=+++
  Bus Selector1 : BusSelector  OutputSignals=electrical.R_0 [Ohm]
  Constant : Constant  Value=ones(SysPara.p,1)  VectorParams1D=off
  Divide : Product  Inputs=*/
  Divide1 : Product  Inputs=*/
  Divide2 : Product  Inputs=*/
  Math Function : Math  Operator=reciprocal  SaturateOnIntegerOverflow=on
  Matrix Sum : Sum  Inputs=+  CollapseMode=Specified dimension
  Matrix Sum1 : Sum  Inputs=+  CollapseMode=Specified dimension
  Matrix Sum2 : Sum  Inputs=+  CollapseMode=Specified dimension
  Product : Product  Multiplication=Matrix(*)
  Subtract : Sum  Inputs=+-
  U_Cell [V] : Outport
  I_Cell [A] : Outport  Port=2
  U_R [V] : Outport  Port=3
  wires:
  Divide/1 -> Matrix Sum1/1
  I_Pack [A]/1 -> Add/2
  Matrix Sum1/1 -> Add/3
  Math Function/1 -> Matrix Sum2/1
  Add/1 -> Divide1/1
  Matrix Sum2/1 -> Divide1/2
  Divide1/1 -> Product/2
  Constant/1 -> Product/1
  Product/1 -> Subtract/1, U_Cell [V]/1  "U_cell [V]"
  Subtract/1 -> Divide2/1, U_R [V]/1  "U_R [V]"
  Divide2/1 -> I_Cell [A]/1  "I_cell [A]"
  Bus Selector1/1 -> Divide/2, Divide2/2, Math Function/1  "<R_0 [Ohm]>"
  Matrix Sum/1 -> Add/1
  I_Balancing_in [A]/1 -> Matrix Sum/1
  U_Potential [V]/1 -> Divide/1, Subtract/2
  BatPara/1 -> Bus Selector1/1

== system sim_battery_system/Battery system simulation/Electrical Submodel/Voltage of battery system ==
  note: Determination of the terminal voltage of the battery pack:
      | 1. Interconnection mechanism of the cells: Cells are first connected in parallel to a group à parallel cell groups are then connected in series
      | 2. Terminal voltage of a parallel cell network corresponds to the individual terminal voltages of the cells in this network.
      | 3. The total voltage of a serial circuit is the sum of its individual voltages.
      | 4. U_Pack (terminal voltage of the battery pack) = sum of the terminal voltages of the serially connected parallel cell composites
  U_Cells [V] : Inport
  Matrix Sum : Sum  Inputs=+
  Multiport Selector : dspindex/Multiport Selector  rowsOrCols=Rows  idxCellArray=1  idxErrMode=Clip Index
  U_Pack [V] : Outport
  wires:
  Matrix Sum/1 -> U_Pack [V]/1  "U_Pack [V]"
  U_Cells [V]/1 -> Multiport Selector/1
  Multiport Selector/1 -> Matrix Sum/1

== system sim_battery_system/Battery system simulation/Electrical Submodel/dt ==
  Clock : Clock
  Subtract : Sum  Inputs=+-
  Unit Delay : UnitDelay  SampleTime=-1
  dt [s] : Outport
  wires:
  Unit Delay/1 -> Subtract/2
  Clock/1 -> Unit Delay/1, Subtract/1
  Subtract/1 -> dt [s]/1

== system sim_battery_system/Battery system simulation/Static and dynamic LIB parameters/LIB Parameter Look-Ups ==
  note: Determination of the current BatPara cell parameter set, dependent on SOC, C-Rate and Temperature of every individual cell of the battery system.
  note: RC-Element 1
  note: RC-Element 2
  note: RC-Element 3
  note: RC-Element 4
  BatState_th_in : Inport
  BatState_el_in : Inport  Port=2
  Apply Deviation Map to C_A : Constant  Value=BatPara.electrical.C_A*SysPara.DeviationMap.C_A  VectorParams1D=off
  Bus Creator : BusCreator  Inputs=10
  Bus Selector : BusSelector  OutputSignals=SOC,I_cell [A]
  Bus Selector1 : BusSelector  OutputSignals=T_cell [°C]
  Divide : Product  Inputs=*/
  Lookup C1 : Lookup_n-D  NumberOfTableDimensions=3  BreakpointsForDimension1=BatPara.electrical.dyn.SOC  BreakpointsForDimension2=BatPara.electrical.dyn.T  BreakpointsForDimension3=BatPara.electrical.dyn.C_rate  BeginIndexSearchUsingPreviousIndexResult=on  Table=BatPara.electrical.dyn.C1  ExtrapMethod=Clip  DiagnosticForOutOfRangeInput=Warning  RemoveProtectionInput=on  UseLastTableValue=on  InternalRulePriority=Speed  RndMeth=Simplest  InputSameDT=on
  Lookup C2 : Lookup_n-D  NumberOfTableDimensions=3  BreakpointsForDimension1=BatPara.electrical.dyn.SOC  BreakpointsForDimension2=BatPara.electrical.dyn.T  BreakpointsForDimension3=BatPara.electrical.dyn.C_rate  BeginIndexSearchUsingPreviousIndexResult=on  Table=BatPara.electrical.dyn.C2  ExtrapMethod=Clip  DiagnosticForOutOfRangeInput=Warning  RemoveProtectionInput=on  UseLastTableValue=on  InternalRulePriority=Speed  RndMeth=Simplest  InputSameDT=on
  Lookup C3 : Lookup_n-D  NumberOfTableDimensions=3  BreakpointsForDimension1=BatPara.electrical.dyn.SOC  BreakpointsForDimension2=BatPara.electrical.dyn.T  BreakpointsForDimension3=BatPara.electrical.dyn.C_rate  BeginIndexSearchUsingPreviousIndexResult=on  Table=BatPara.electrical.dyn.C3  ExtrapMethod=Clip  DiagnosticForOutOfRangeInput=Warning  RemoveProtectionInput=on  UseLastTableValue=on  InternalRulePriority=Speed  RndMeth=Simplest  InputSameDT=on
  Lookup C4 : Lookup_n-D  NumberOfTableDimensions=3  BreakpointsForDimension1=BatPara.electrical.dyn.SOC  BreakpointsForDimension2=BatPara.electrical.dyn.T  BreakpointsForDimension3=BatPara.electrical.dyn.C_rate  BeginIndexSearchUsingPreviousIndexResult=on  Table=BatPara.electrical.dyn.C4  ExtrapMethod=Clip  DiagnosticForOutOfRangeInput=Warning  RemoveProtectionInput=on  UseLastTableValue=on  InternalRulePriority=Speed  RndMeth=Simplest  InputSameDT=on
  Lookup R1 : Lookup_n-D  NumberOfTableDimensions=3  BreakpointsForDimension1=BatPara.electrical.dyn.SOC  BreakpointsForDimension2=BatPara.electrical.dyn.T  BreakpointsForDimension3=BatPara.electrical.dyn.C_rate  BeginIndexSearchUsingPreviousIndexResult=on  Table=BatPara.electrical.dyn.R1  ExtrapMethod=Clip  DiagnosticForOutOfRangeInput=Warning  RemoveProtectionInput=on  UseLastTableValue=on  InternalRulePriority=Speed  RndMeth=Simplest  InputSameDT=on
  Lookup R2 : Lookup_n-D  NumberOfTableDimensions=3  BreakpointsForDimension1=BatPara.electrical.dyn.SOC  BreakpointsForDimension2=BatPara.electrical.dyn.T  BreakpointsForDimension3=BatPara.electrical.dyn.C_rate  BeginIndexSearchUsingPreviousIndexResult=on  Table=BatPara.electrical.dyn.R2  ExtrapMethod=Clip  DiagnosticForOutOfRangeInput=Warning  RemoveProtectionInput=on  UseLastTableValue=on  InternalRulePriority=Speed  RndMeth=Simplest  InputSameDT=on
  Lookup R3 : Lookup_n-D  NumberOfTableDimensions=3  BreakpointsForDimension1=BatPara.electrical.dyn.SOC  BreakpointsForDimension2=BatPara.electrical.dyn.T  BreakpointsForDimension3=BatPara.electrical.dyn.C_rate  BeginIndexSearchUsingPreviousIndexResult=on  Table=BatPara.electrical.dyn.R3  ExtrapMethod=Clip  DiagnosticForOutOfRangeInput=Warning  RemoveProtectionInput=on  UseLastTableValue=on  InternalRulePriority=Speed  RndMeth=Simplest  InputSameDT=on
  Lookup R4 : Lookup_n-D  NumberOfTableDimensions=3  BreakpointsForDimension1=BatPara.electrical.dyn.SOC  BreakpointsForDimension2=BatPara.electrical.dyn.T  BreakpointsForDimension3=BatPara.electrical.dyn.C_rate  BeginIndexSearchUsingPreviousIndexResult=on  Table=BatPara.electrical.dyn.R4  ExtrapMethod=Clip  DiagnosticForOutOfRangeInput=Warning  RemoveProtectionInput=on  UseLastTableValue=on  InternalRulePriority=Speed  RndMeth=Simplest  InputSameDT=on
  Lookup R_0 : Lookup_n-D  NumberOfTableDimensions=3  BreakpointsForDimension1=BatPara.electrical.dyn.SOC  BreakpointsForDimension2=BatPara.electrical.dyn.T  BreakpointsForDimension3=BatPara.electrical.dyn.C_rate  BeginIndexSearchUsingPreviousIndexResult=on  Table=BatPara.electrical.dyn.R_0  ExtrapMethod=Clip  DiagnosticForOutOfRangeInput=Warning  RemoveProtectionInput=on  UseLastTableValue=on  InternalRulePriority=Speed  RndMeth=Simplest  InputSameDT=on
  BatPara_el_uniform : Outport
  wires:
  Bus Selector/1 -> Lookup R_0/1, Lookup R1/1, Lookup C1/1, Lookup C4/1, Lookup R4/1, Lookup C3/1, Lookup R3/1, Lookup C2/1, Lookup R2/1  "<SOC>"
  Divide/1 -> Lookup R_0/2, Lookup R1/2, Lookup C1/2, Lookup C4/2, Lookup R4/2, Lookup C3/2, Lookup R3/2, Lookup C2/2, Lookup R2/2
  Lookup R_0/1 -> Bus Creator/1  "R_0 [Ohm]"
  Bus Selector1/1 -> Lookup R3/3, Lookup C3/3, Lookup R4/3, Lookup C4/3, Lookup R_0/3, Lookup R1/3, Lookup C1/3, Lookup R2/3, Lookup C2/3  "<T_cell [°C]>"
  Lookup R1/1 -> Bus Creator/2  "R1 [Ohm]"
  Lookup R2/1 -> Bus Creator/4  "R2 [Ohm]"
  Lookup C1/1 -> Bus Creator/3  "C1 [F]"
  Lookup C2/1 -> Bus Creator/5  "C2 [F]"
  BatState_el_in/1 -> Bus Selector/1
  Apply Deviation Map to C_A/1 -> Divide/2, Bus Creator/10  "C_A [Ah]"
  Bus Creator/1 -> BatPara_el_uniform/1
  Bus Selector/2 -> Divide/1  "<I_cell [A]>"
  BatState_th_in/1 -> Bus Selector1/1
  Lookup C4/1 -> Bus Creator/9  "C4 [F]"
  Lookup C3/1 -> Bus Creator/7  "C3 [F]"
  Lookup R4/1 -> Bus Creator/8  "R4 [Ohm]"
  Lookup R3/1 -> Bus Creator/6  "R3 [Ohm]"

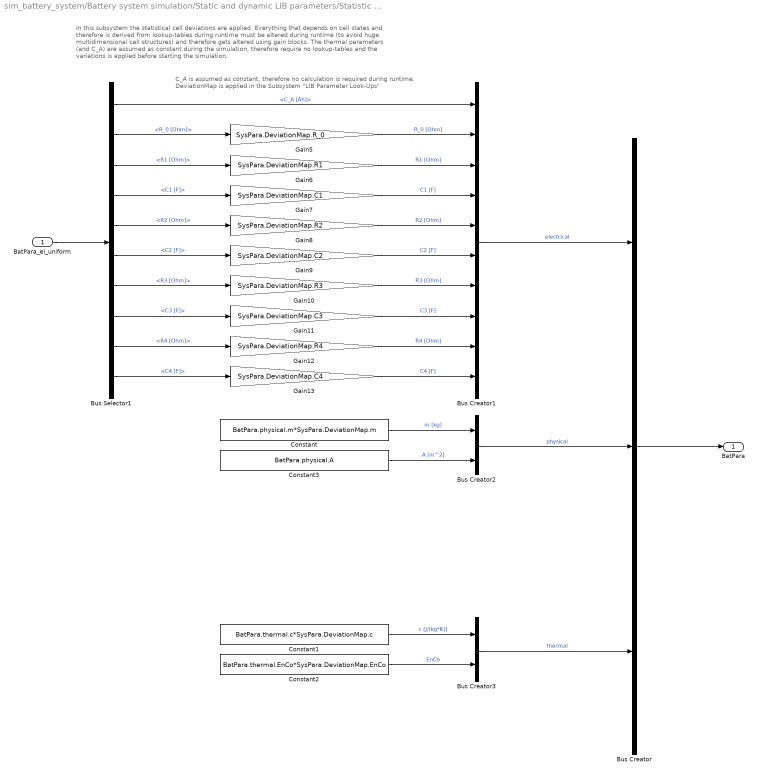
== system sim_battery_system/Battery system simulation/Static and dynamic LIB parameters/Statistic Cell Deviations ==
  note: In this subsystem the statistical cell deviations are applied. Everything that depends on cell states and therefore is derived from lookup-tables during runtime
      | must be altered during runtime (to avoid huge multidimensional cell structures) and therefore gets altered using gain blocks. The thermal parameters (and C_A)
      | are assumed as constant during the simulation, therefore require no lookup-tables and the variations is applied before starting the simulation.
  note: C_A is assumed as constant, therefore no calculation is required during runtime.
      | DeviationMap is applied in the Subsystem "LIB Parameter Look-Ups"
  "BatPara_el_uniform " : Inport
  Bus Creator : BusCreator  Inputs=3
  Bus Creator1 : BusCreator  Inputs=10
  Bus Creator2 : BusCreator  Inputs=2
  Bus Creator3 : BusCreator  Inputs=2
  Bus Selector1 : BusSelector  OutputSignals=C_A [Ah],R_0 [Ohm],R1 [Ohm],C1 [F],R2 [Ohm],C2 [F],R3 [Ohm],C3 [F],R4 [Ohm],C4 [F]
  Constant : Constant  Value=BatPara.physical.m*SysPara.DeviationMap.m
  Constant1 : Constant  Value=BatPara.thermal.c*SysPara.DeviationMap.c
  Constant2 : Constant  Value=BatPara.thermal.EnCo*SysPara.DeviationMap.EnCo
  Constant3 : Constant  Value=BatPara.physical.A
  Gain10 : Gain  Gain=SysPara.DeviationMap.R3
  Gain11 : Gain  Gain=SysPara.DeviationMap.C3
  Gain12 : Gain  Gain=SysPara.DeviationMap.R4
  Gain13 : Gain  Gain=SysPara.DeviationMap.C4
  Gain5 : Gain  Gain=SysPara.DeviationMap.R_0
  Gain6 : Gain  Gain=SysPara.DeviationMap.R1
  Gain7 : Gain  Gain=SysPara.DeviationMap.C1
  Gain8 : Gain  Gain=SysPara.DeviationMap.R2
  Gain9 : Gain  Gain=SysPara.DeviationMap.C2
  BatPara : Outport
  wires:
  "BatPara_el_uniform "/1 -> Bus Selector1/1
  Bus Selector1/2 -> Gain5/1  "<R_0 [Ohm]>"
  Bus Selector1/3 -> Gain6/1  "<R1 [Ohm]>"
  Bus Selector1/4 -> Gain7/1  "<C1 [F]>"
  Bus Selector1/5 -> Gain8/1  "<R2 [Ohm]>"
  Bus Selector1/6 -> Gain9/1  "<C2 [F]>"
  Bus Selector1/7 -> Gain10/1  "<R3 [Ohm]>"
  Bus Selector1/8 -> Gain11/1  "<C3 [F]>"
  Bus Selector1/9 -> Gain12/1  "<R4 [Ohm]>"
  Bus Selector1/10 -> Gain13/1  "<C4 [F]>"
  Bus Selector1/1 -> Bus Creator1/1  "<C_A [Ah]>"
  Gain5/1 -> Bus Creator1/2  "R_0 [Ohm]"
  Gain6/1 -> Bus Creator1/3  "R1 [Ohm]"
  Gain7/1 -> Bus Creator1/4  "C1 [F]"
  Gain8/1 -> Bus Creator1/5  "R2 [Ohm]"
  Gain9/1 -> Bus Creator1/6  "C2 [F]"
  Gain10/1 -> Bus Creator1/7  "R3 [Ohm]"
  Gain11/1 -> Bus Creator1/8  "C3 [F]"
  Gain12/1 -> Bus Creator1/9  "R4 [Ohm]"
  Gain13/1 -> Bus Creator1/10  "C4 [F]"
  Bus Creator1/1 -> Bus Creator/1  "electrical"
  Bus Creator2/1 -> Bus Creator/2  "physical"
  Constant/1 -> Bus Creator2/1  "m [kg]"
  Constant1/1 -> Bus Creator3/1  "c [J/(kg*K)]"
  Constant2/1 -> Bus Creator3/2  "EnCo"
  Constant3/1 -> Bus Creator2/2  "A [m^2]"
  Bus Creator/1 -> BatPara/1
  Bus Creator3/1 -> Bus Creator/3  "thermal"
